simulink model "EPT"  (R2019b)
settings: Solver=FixedStepDiscrete  StartTime=0.0  StopTime=5  FixedStep=0.005  RelTol=1e-3  EnableMultiTasking=on
PreLoadFcn:
  | try, model_open; catch, disp('Error occurred while executing model pre-load callback: model_open.m'); disp('Please assure that the MATLAB working directory is set to the model directory before opening.'); end
InitFcn:
  | try, model_open; catch, end
undefined symbols (not defined in the file or in its folder): Bridge, GCM, H, ln, raptor_get_param_eval, raptor_get_safe_string, raptor_xcp_function
libraries: Raptor_lib x2810, simulink x374, hdlsllib x19
(part 30 of 45)

== system EPT/Foreground_TimeBase_5ms/CAN/CAN3_exec/HyPer9_MCU/TPDO2/Convert_Byte2Data3 ==
  LowByte : Inport
  HighByte : Inport  Port=2
  Offset : Inport  Port=3
  Factor : Inport  Port=4
  Add2 : Sum
  Add5 : Sum
  Compare To Zero : simulink/Logic and Bit Operations/Compare To Zero  relop===  OutDataTypeStr=boolean
  Constant1 : Constant
  Constant10 : Constant  Value=256
  Data Type Conversion1 : DataTypeConversion  OutDataTypeStr=int16
  Data Type Conversion10 : DataTypeConversion  OutDataTypeStr=double
  Divide6 : Product  Inputs=**
  Divide9 : Product  Inputs=**
  Switch : Switch  Criteria=u2 > Threshold
  Data : Outport  VectorParamsAs1DForOutWhenUnconnected=off
  wires:
  Constant1/1 -> Switch/1
  Factor/1 -> Compare To Zero/1, Switch/3
  Compare To Zero/1 -> Switch/2
  Switch/1 -> Divide9/2
  Divide6/1 -> Add2/2
  Add5/1 -> Data Type Conversion10/1
  Constant10/1 -> Divide6/2
  Divide9/1 -> Add5/1
  Add2/1 -> Data Type Conversion1/1
  Data Type Conversion10/1 -> Data/1
  Offset/1 -> Add5/2
  HighByte/1 -> Divide6/1
  LowByte/1 -> Add2/1
  Data Type Conversion1/1 -> Divide9/1

== system EPT/Foreground_TimeBase_5ms/CAN/CAN3_exec/HyPer9_MCU/TPDO3/Byte6 ==
  Byte : Inport
  Bitwise AND : simulink/Logic and Bit Operations/Bitwise Operator  logicop=AND  UseBitMask=on  BitMask=bin2dec('10')  BitMaskRealWorld=Stored Integer
  Bitwise AND1 : simulink/Logic and Bit Operations/Bitwise Operator  logicop=AND  UseBitMask=on  BitMask=bin2dec('100')  BitMaskRealWorld=Stored Integer
  Bitwise AND2 : simulink/Logic and Bit Operations/Bitwise Operator  logicop=AND  UseBitMask=on  BitMask=bin2dec('1000')  BitMaskRealWorld=Stored Integer
  Bitwise AND3 : simulink/Logic and Bit Operations/Bitwise Operator  logicop=AND  UseBitMask=on  BitMask=bin2dec('10000000')  BitMaskRealWorld=Stored Integer
  Bitwise AND7 : simulink/Logic and Bit Operations/Bitwise Operator  logicop=AND  UseBitMask=on  BitMask=bin2dec('1')  BitMaskRealWorld=Stored Integer
  IsPositive{,1..4} (5 alike) : simulink/Logic and Bit Operations/Compare To Zero  relop=>  OutDataTypeStr=boolean
  Digital Input 17 State : Outport
  Digital Input 18 State : Outport  Port=2
  Digital Input 19 State : Outport  Port=3
  "Toggle bit " : Outport  Port=4
  Driver Output 4 - State : Outport  Port=5
  wires:
  Bitwise AND7/1 -> IsPositive/1
  Bitwise AND3/1 -> IsPositive4/1
  Byte/1 -> Bitwise AND7/1, Bitwise AND1/1, Bitwise AND2/1, Bitwise AND3/1, Bitwise AND/1
  Bitwise AND/1 -> IsPositive1/1
  Bitwise AND2/1 -> IsPositive3/1
  Bitwise AND1/1 -> IsPositive2/1
  IsPositive/1 -> Digital Input 17 State/1
  IsPositive1/1 -> Digital Input 18 State/1
  IsPositive2/1 -> Digital Input 19 State/1
  IsPositive3/1 -> "Toggle bit "/1
  IsPositive4/1 -> Driver Output 4 - State/1

== system EPT/Foreground_TimeBase_5ms/CAN/CAN3_exec/HyPer9_MCU/TPDO3/Byte7 ==
  Byte : Inport
  Bit Shift : hdlsllib/Logic and Bit Operations/Bit Shift  mode=Shift Right Logical  N=5
  Bitwise AND : simulink/Logic and Bit Operations/Bitwise Operator  logicop=AND  UseBitMask=on  BitMask=bin2dec('10')  BitMaskRealWorld=Stored Integer
  Bitwise AND1 : simulink/Logic and Bit Operations/Bitwise Operator  logicop=AND  UseBitMask=on  BitMask=bin2dec('100')  BitMaskRealWorld=Stored Integer
  Bitwise AND2 : simulink/Logic and Bit Operations/Bitwise Operator  logicop=AND  UseBitMask=on  BitMask=bin2dec('1000')  BitMaskRealWorld=Stored Integer
  Bitwise AND3 : simulink/Logic and Bit Operations/Bitwise Operator  logicop=AND  UseBitMask=on  BitMask=bin2dec('10000')  BitMaskRealWorld=Stored Integer
  Bitwise AND4 : simulink/Logic and Bit Operations/Bitwise Operator  logicop=AND  UseBitMask=on  BitMask=bin2dec('11100000')  BitMaskRealWorld=Stored Integer
  Bitwise AND7 : simulink/Logic and Bit Operations/Bitwise Operator  logicop=AND  UseBitMask=on  BitMask=bin2dec('1')  BitMaskRealWorld=Stored Integer
  IsPositive{,1..4} (5 alike) : simulink/Logic and Bit Operations/Compare To Zero  relop=>  OutDataTypeStr=boolean
  Driver Output 1 - State : Outport
  Driver Output 2 - State : Outport  Port=2
  Driver Output 3 - State : Outport  Port=3
  Digital Output 1 - State : Outport  Port=4
  Digital Output 2 - State : Outport  Port=5
  "Fault Level " : Outport  Port=6
  wires:
  Bitwise AND1/1 -> IsPositive2/1
  Bitwise AND2/1 -> IsPositive3/1
  Bitwise AND/1 -> IsPositive1/1
  Bitwise AND4/1 -> Bit Shift/1
  Byte/1 -> Bitwise AND/1, Bitwise AND4/1, Bitwise AND3/1, Bitwise AND2/1, Bitwise AND1/1, Bitwise AND7/1
  Bitwise AND3/1 -> IsPositive4/1
  Bitwise AND7/1 -> IsPositive/1
  Bit Shift/1 -> "Fault Level "/1
  IsPositive/1 -> Driver Output 1 - State/1
  IsPositive1/1 -> Driver Output 2 - State/1
  IsPositive2/1 -> Driver Output 3 - State/1
  IsPositive3/1 -> Digital Output 1 - State/1
  IsPositive4/1 -> Digital Output 2 - State/1

== system EPT/Foreground_TimeBase_5ms/CAN/CAN3_exec/HyPer9_MCU/TPDO3/Convert_Byte2Data ==
  LowByte : Inport
  HighByte : Inport  Port=2
  Offset : Inport  Port=3
  Factor : Inport  Port=4
  Add2 : Sum
  Add5 : Sum
  Compare To Zero : simulink/Logic and Bit Operations/Compare To Zero  relop===  OutDataTypeStr=boolean
  Constant1 : Constant
  Constant10 : Constant  Value=256
  Data Type Conversion1 : DataTypeConversion  OutDataTypeStr=int16
  Data Type Conversion10 : DataTypeConversion  OutDataTypeStr=double
  Divide6 : Product  Inputs=**
  Divide9 : Product  Inputs=**
  Switch : Switch  Criteria=u2 > Threshold
  Data : Outport  VectorParamsAs1DForOutWhenUnconnected=off
  wires:
  Constant1/1 -> Switch/1
  Factor/1 -> Compare To Zero/1, Switch/3
  Compare To Zero/1 -> Switch/2
  Switch/1 -> Divide9/2
  Divide6/1 -> Add2/2
  Add5/1 -> Data Type Conversion10/1
  Constant10/1 -> Divide6/2
  Divide9/1 -> Add5/1
  Add2/1 -> Data Type Conversion1/1
  Data Type Conversion10/1 -> Data/1
  Offset/1 -> Add5/2
  HighByte/1 -> Divide6/1
  LowByte/1 -> Add2/1
  Data Type Conversion1/1 -> Divide9/1

== system EPT/Foreground_TimeBase_5ms/CAN/CAN3_exec/HyPer9_MCU/TPDO3/Convert_Byte2Data1 ==
  LowByte : Inport
  HighByte : Inport  Port=2
  Offset : Inport  Port=3
  Factor : Inport  Port=4
  Add2 : Sum
  Add5 : Sum
  Compare To Zero : simulink/Logic and Bit Operations/Compare To Zero  relop===  OutDataTypeStr=boolean
  Constant1 : Constant
  Constant10 : Constant  Value=256
  Data Type Conversion1 : DataTypeConversion  OutDataTypeStr=int16
  Data Type Conversion10 : DataTypeConversion  OutDataTypeStr=double
  Divide6 : Product  Inputs=**
  Divide9 : Product  Inputs=**
  Switch : Switch  Criteria=u2 > Threshold
  Data : Outport  VectorParamsAs1DForOutWhenUnconnected=off
  wires:
  Data Type Conversion1/1 -> Divide9/1
  LowByte/1 -> Add2/1
  HighByte/1 -> Divide6/1
  Offset/1 -> Add5/2
  Data Type Conversion10/1 -> Data/1
  Add2/1 -> Data Type Conversion1/1
  Divide9/1 -> Add5/1
  Constant10/1 -> Divide6/2
  Add5/1 -> Data Type Conversion10/1
  Divide6/1 -> Add2/2
  Switch/1 -> Divide9/2
  Compare To Zero/1 -> Switch/2
  Factor/1 -> Switch/3, Compare To Zero/1
  Constant1/1 -> Switch/1

== system EPT/Foreground_TimeBase_5ms/CAN/CAN3_exec/HyPer9_MCU/TPDO3/Digital Input 1 to 8 - State ==
  Byte : Inport
  Bitwise AND : simulink/Logic and Bit Operations/Bitwise Operator  logicop=AND  UseBitMask=on  BitMask=bin2dec('10')  BitMaskRealWorld=Stored Integer
  Bitwise AND1 : simulink/Logic and Bit Operations/Bitwise Operator  logicop=AND  UseBitMask=on  BitMask=bin2dec('100')  BitMaskRealWorld=Stored Integer
  Bitwise AND2 : simulink/Logic and Bit Operations/Bitwise Operator  logicop=AND  UseBitMask=on  BitMask=bin2dec('1000')  BitMaskRealWorld=Stored Integer
  Bitwise AND3 : simulink/Logic and Bit Operations/Bitwise Operator  logicop=AND  UseBitMask=on  BitMask=bin2dec('10000')  BitMaskRealWorld=Stored Integer
  Bitwise AND4 : simulink/Logic and Bit Operations/Bitwise Operator  logicop=AND  UseBitMask=on  BitMask=bin2dec('100000')  BitMaskRealWorld=Stored Integer
  Bitwise AND5 : simulink/Logic and Bit Operations/Bitwise Operator  logicop=AND  UseBitMask=on  BitMask=bin2dec('1000000')  BitMaskRealWorld=Stored Integer
  Bitwise AND6 : simulink/Logic and Bit Operations/Bitwise Operator  logicop=AND  UseBitMask=on  BitMask=bin2dec('10000000')  BitMaskRealWorld=Stored Integer
  Bitwise AND7 : simulink/Logic and Bit Operations/Bitwise Operator  logicop=AND  UseBitMask=on  BitMask=bin2dec('1')  BitMaskRealWorld=Stored Integer
  IsPositive{,1..7} (8 alike) : simulink/Logic and Bit Operations/Compare To Zero  relop=>  OutDataTypeStr=boolean
  Digital Input 1 State : Outport
  Digital Input 2 State : Outport  Port=2
  Digital Input 3 State : Outport  Port=3
  Digital Input 4 State : Outport  Port=4
  Digital Input 5 State : Outport  Port=5
  Digital Input 6 State : Outport  Port=6
  Digital Input 7 State : Outport  Port=7
  Digital Input 8 State : Outport  Port=8
  wires:
  Bitwise AND1/1 -> IsPositive2/1
  Bitwise AND2/1 -> IsPositive3/1
  Bitwise AND/1 -> IsPositive1/1
  Bitwise AND4/1 -> IsPositive5/1
  Byte/1 -> Bitwise AND/1, Bitwise AND6/1, Bitwise AND5/1, Bitwise AND4/1, Bitwise AND3/1, Bitwise AND2/1, Bitwise AND1/1, Bitwise AND7/1
  Bitwise AND3/1 -> IsPositive4/1
  Bitwise AND6/1 -> IsPositive7/1
  Bitwise AND5/1 -> IsPositive6/1
  Bitwise AND7/1 -> IsPositive/1
  IsPositive/1 -> Digital Input 1 State/1
  IsPositive1/1 -> Digital Input 2 State/1
  IsPositive2/1 -> Digital Input 3 State/1
  IsPositive3/1 -> Digital Input 4 State/1
  IsPositive4/1 -> Digital Input 5 State/1
  IsPositive5/1 -> Digital Input 6 State/1
  IsPositive6/1 -> Digital Input 7 State/1
  IsPositive7/1 -> Digital Input 8 State/1

== system EPT/Foreground_TimeBase_5ms/CAN/CAN3_exec/HyPer9_MCU/TPDO3/Digital Input 9 to 16 - State ==
  Byte : Inport
  Bitwise AND : simulink/Logic and Bit Operations/Bitwise Operator  logicop=AND  UseBitMask=on  BitMask=bin2dec('10')  BitMaskRealWorld=Stored Integer
  Bitwise AND1 : simulink/Logic and Bit Operations/Bitwise Operator  logicop=AND  UseBitMask=on  BitMask=bin2dec('100')  BitMaskRealWorld=Stored Integer
  Bitwise AND2 : simulink/Logic and Bit Operations/Bitwise Operator  logicop=AND  UseBitMask=on  BitMask=bin2dec('1000')  BitMaskRealWorld=Stored Integer
  Bitwise AND3 : simulink/Logic and Bit Operations/Bitwise Operator  logicop=AND  UseBitMask=on  BitMask=bin2dec('10000')  BitMaskRealWorld=Stored Integer
  Bitwise AND4 : simulink/Logic and Bit Operations/Bitwise Operator  logicop=AND  UseBitMask=on  BitMask=bin2dec('100000')  BitMaskRealWorld=Stored Integer
  Bitwise AND5 : simulink/Logic and Bit Operations/Bitwise Operator  logicop=AND  UseBitMask=on  BitMask=bin2dec('1000000')  BitMaskRealWorld=Stored Integer
  Bitwise AND6 : simulink/Logic and Bit Operations/Bitwise Operator  logicop=AND  UseBitMask=on  BitMask=bin2dec('10000000')  BitMaskRealWorld=Stored Integer
  Bitwise AND7 : simulink/Logic and Bit Operations/Bitwise Operator  logicop=AND  UseBitMask=on  BitMask=bin2dec('1')  BitMaskRealWorld=Stored Integer
  IsPositive{,1..7} (8 alike) : simulink/Logic and Bit Operations/Compare To Zero  relop=>  OutDataTypeStr=boolean
  Digital Input 9 State : Outport
  Digital Input 10 State : Outport  Port=2
  Digital Input 11 State : Outport  Port=3
  Digital Input 12 State : Outport  Port=4
  Digital Input 13 State : Outport  Port=5
  Digital Input 14 State : Outport  Port=6
  Digital Input 15 State : Outport  Port=7
  Digital Input 16 State : Outport  Port=8
  wires:
  Bitwise AND7/1 -> IsPositive/1
  Bitwise AND5/1 -> IsPositive6/1
  Bitwise AND6/1 -> IsPositive7/1
  Bitwise AND3/1 -> IsPositive4/1
  Byte/1 -> Bitwise AND7/1, Bitwise AND1/1, Bitwise AND2/1, Bitwise AND3/1, Bitwise AND4/1, Bitwise AND5/1, Bitwise AND6/1, Bitwise AND/1
  Bitwise AND4/1 -> IsPositive5/1
  Bitwise AND/1 -> IsPositive1/1
  Bitwise AND2/1 -> IsPositive3/1
  Bitwise AND1/1 -> IsPositive2/1
  IsPositive/1 -> Digital Input 9 State/1
  IsPositive1/1 -> Digital Input 10 State/1
  IsPositive2/1 -> Digital Input 11 State/1
  IsPositive3/1 -> Digital Input 12 State/1
  IsPositive4/1 -> Digital Input 13 State/1
  IsPositive5/1 -> Digital Input 14 State/1
  IsPositive6/1 -> Digital Input 15 State/1
  IsPositive7/1 -> Digital Input 16 State/1

== system EPT/Foreground_TimeBase_5ms/CAN/CAN3_exec/HyPer9_MCU/TPDO4/Byte6 ==
  Byte : Inport
  Bitwise AND : simulink/Logic and Bit Operations/Bitwise Operator  logicop=AND  UseBitMask=on  BitMask=bin2dec('100')  BitMaskRealWorld=Stored Integer
  Bitwise AND1 : simulink/Logic and Bit Operations/Bitwise Operator  logicop=AND  UseBitMask=on  BitMask=bin2dec('1000')  BitMaskRealWorld=Stored Integer
  Bitwise AND2 : simulink/Logic and Bit Operations/Bitwise Operator  logicop=AND  UseBitMask=on  BitMask=bin2dec('10000')  BitMaskRealWorld=Stored Integer
  Bitwise AND3 : simulink/Logic and Bit Operations/Bitwise Operator  logicop=AND  UseBitMask=on  BitMask=bin2dec('100000')  BitMaskRealWorld=Stored Integer
  Bitwise AND4 : simulink/Logic and Bit Operations/Bitwise Operator  logicop=AND  UseBitMask=on  BitMask=bin2dec('1000000')  BitMaskRealWorld=Stored Integer
  Bitwise AND7 : simulink/Logic and Bit Operations/Bitwise Operator  logicop=AND  UseBitMask=on  BitMask=bin2dec('11')  BitMaskRealWorld=Stored Integer
  IsPositive{1..5} (5 alike) : simulink/Logic and Bit Operations/Compare To Zero  relop=>  OutDataTypeStr=boolean
  Motor 1 - Control Mode : Outport
  Motor 1 - PWM Output : Outport  Port=2
  Motor 1 - Reference Speed/Torque : Outport  Port=3
  Motor 1 - Emergency Stop : Outport  Port=4
  Motor 1 - Safe Stop : Outport  Port=5
  Motor 1 - Speed Limit : Outport  Port=6
  wires:
  IsPositive4/1 -> Motor 1 - Safe Stop/1
  IsPositive3/1 -> Motor 1 - Emergency Stop/1
  IsPositive2/1 -> Motor 1 - Reference Speed/Torque/1
  IsPositive1/1 -> Motor 1 - PWM Output/1
  Bitwise AND7/1 -> Motor 1 - Control Mode/1
  Bitwise AND1/1 -> IsPositive2/1
  Bitwise AND2/1 -> IsPositive3/1
  Bitwise AND/1 -> IsPositive1/1
  Byte/1 -> Bitwise AND/1, Bitwise AND4/1, Bitwise AND3/1, Bitwise AND2/1, Bitwise AND1/1, Bitwise AND7/1
  Bitwise AND3/1 -> IsPositive4/1
  Bitwise AND4/1 -> IsPositive5/1
  IsPositive5/1 -> Motor 1 - Speed Limit/1

== system EPT/Foreground_TimeBase_5ms/CAN/CAN3_exec/HyPer9_MCU/TPDO4/Convert_Byte2Data ==
  LowByte : Inport
  HighByte : Inport  Port=2
  Offset : Inport  Port=3
  Factor : Inport  Port=4
  Add2 : Sum
  Add5 : Sum
  Compare To Zero : simulink/Logic and Bit Operations/Compare To Zero  relop===  OutDataTypeStr=boolean
  Constant1 : Constant
  Constant10 : Constant  Value=256
  Data Type Conversion1 : DataTypeConversion  OutDataTypeStr=int16
  Data Type Conversion10 : DataTypeConversion  OutDataTypeStr=double
  Divide6 : Product  Inputs=**
  Divide9 : Product  Inputs=**
  Switch : Switch  Criteria=u2 > Threshold
  Data : Outport  VectorParamsAs1DForOutWhenUnconnected=off
  wires:
  Data Type Conversion1/1 -> Divide9/1
  LowByte/1 -> Add2/1
  HighByte/1 -> Divide6/1
  Offset/1 -> Add5/2
  Data Type Conversion10/1 -> Data/1
  Add2/1 -> Data Type Conversion1/1
  Divide9/1 -> Add5/1
  Constant10/1 -> Divide6/2
  Add5/1 -> Data Type Conversion10/1
  Divide6/1 -> Add2/2
  Switch/1 -> Divide9/2
  Compare To Zero/1 -> Switch/2
  Factor/1 -> Switch/3, Compare To Zero/1
  Constant1/1 -> Switch/1

== system EPT/Foreground_TimeBase_5ms/CAN/CAN3_exec/HyPer9_MCU/TPDO4/Convert_Byte2Data1 ==
  LowByte : Inport
  HighByte : Inport  Port=2
  Offset : Inport  Port=3
  Factor : Inport  Port=4
  Add2 : Sum
  Add5 : Sum
  Compare To Zero : simulink/Logic and Bit Operations/Compare To Zero  relop===  OutDataTypeStr=boolean
  Constant1 : Constant
  Constant10 : Constant  Value=256
  Data Type Conversion1 : DataTypeConversion  OutDataTypeStr=int16
  Data Type Conversion10 : DataTypeConversion  OutDataTypeStr=double
  Divide6 : Product  Inputs=**
  Divide9 : Product  Inputs=**
  Switch : Switch  Criteria=u2 > Threshold
  Data : Outport  VectorParamsAs1DForOutWhenUnconnected=off
  wires:
  Constant1/1 -> Switch/1
  Factor/1 -> Compare To Zero/1, Switch/3
  Compare To Zero/1 -> Switch/2
  Switch/1 -> Divide9/2
  Divide6/1 -> Add2/2
  Add5/1 -> Data Type Conversion10/1
  Constant10/1 -> Divide6/2
  Divide9/1 -> Add5/1
  Add2/1 -> Data Type Conversion1/1
  Data Type Conversion10/1 -> Data/1
  Offset/1 -> Add5/2
  HighByte/1 -> Divide6/1
  LowByte/1 -> Add2/1
  Data Type Conversion1/1 -> Divide9/1

== system EPT/Foreground_TimeBase_5ms/CAN/CAN3_exec/HyPer9_MCU/TPDO4/Convert_Byte2Data2 ==
  Offset : Inport
  LowByte : Inport  Port=2
  Factor : Inport  Port=3
  Add5 : Sum
  Compare To Zero : simulink/Logic and Bit Operations/Compare To Zero  relop===  OutDataTypeStr=boolean
  Constant1 : Constant
  Data Type Conversion1 : DataTypeConversion  OutDataTypeStr=uint8
  Data Type Conversion10 : DataTypeConversion  OutDataTypeStr=double
  Divide9 : Product  Inputs=**
  Switch : Switch  Criteria=u2 > Threshold
  Data : Outport  VectorParamsAs1DForOutWhenUnconnected=off
  wires:
  Data Type Conversion10/1 -> Data/1
  Offset/1 -> Add5/2
  Compare To Zero/1 -> Switch/2
  Data Type Conversion1/1 -> Divide9/1
  Add5/1 -> Data Type Conversion10/1
  Divide9/1 -> Add5/1
  Switch/1 -> Divide9/2
  Constant1/1 -> Switch/1
  Factor/1 -> Compare To Zero/1, Switch/3
  LowByte/1 -> Data Type Conversion1/1

== system EPT/Foreground_TimeBase_5ms/CAN/CAN3_exec/HyPer9_MCU/TPDO4/Convert_Byte2Data3 ==
  Offset : Inport
  LowByte : Inport  Port=2
  Factor : Inport  Port=3
  Add5 : Sum
  Compare To Zero : simulink/Logic and Bit Operations/Compare To Zero  relop===  OutDataTypeStr=boolean
  Constant1 : Constant
  Data Type Conversion1 : DataTypeConversion  OutDataTypeStr=uint8
  Data Type Conversion10 : DataTypeConversion  OutDataTypeStr=double
  Divide9 : Product  Inputs=**
  Switch : Switch  Criteria=u2 > Threshold
  Data : Outport  VectorParamsAs1DForOutWhenUnconnected=off
  wires:
  LowByte/1 -> Data Type Conversion1/1
  Factor/1 -> Switch/3, Compare To Zero/1
  Constant1/1 -> Switch/1
  Switch/1 -> Divide9/2
  Divide9/1 -> Add5/1
  Add5/1 -> Data Type Conversion10/1
  Data Type Conversion1/1 -> Divide9/1
  Compare To Zero/1 -> Switch/2
  Offset/1 -> Add5/2
  Data Type Conversion10/1 -> Data/1

== system EPT/Foreground_TimeBase_5ms/CAN/CAN3_exec/HyPer9_MCU/TPDO4/Motor 1 - State ==
  Byte : Inport
  Bitwise AND7 : simulink/Logic and Bit Operations/Bitwise Operator  logicop=AND  UseBitMask=on  BitMask=bin2dec('1111')  BitMaskRealWorld=Stored Integer
  Motor 1 - State : Outport
  wires:
  Bitwise AND7/1 -> Motor 1 - State/1
  Byte/1 -> Bitwise AND7/1

== system EPT/Foreground_TimeBase_5ms/CAN/CAN3_exec/HyPer9_MCU/TPDO5/Byte6 ==
  Byte : Inport
  Bitwise AND : simulink/Logic and Bit Operations/Bitwise Operator  logicop=AND  UseBitMask=on  BitMask=bin2dec('100')  BitMaskRealWorld=Stored Integer
  Bitwise AND1 : simulink/Logic and Bit Operations/Bitwise Operator  logicop=AND  UseBitMask=on  BitMask=bin2dec('1000')  BitMaskRealWorld=Stored Integer
  Bitwise AND2 : simulink/Logic and Bit Operations/Bitwise Operator  logicop=AND  UseBitMask=on  BitMask=bin2dec('10000')  BitMaskRealWorld=Stored Integer
  Bitwise AND3 : simulink/Logic and Bit Operations/Bitwise Operator  logicop=AND  UseBitMask=on  BitMask=bin2dec('100000')  BitMaskRealWorld=Stored Integer
  Bitwise AND4 : simulink/Logic and Bit Operations/Bitwise Operator  logicop=AND  UseBitMask=on  BitMask=bin2dec('1000000')  BitMaskRealWorld=Stored Integer
  Bitwise AND7 : simulink/Logic and Bit Operations/Bitwise Operator  logicop=AND  UseBitMask=on  BitMask=bin2dec('11')  BitMaskRealWorld=Stored Integer
  IsPositive{1..5} (5 alike) : simulink/Logic and Bit Operations/Compare To Zero  relop=>  OutDataTypeStr=boolean
  Motor 2 - Control Mode : Outport
  Motor 2 - PWM Output : Outport  Port=2
  Motor 2 - Reference Speed/Torque : Outport  Port=3
  Motor 2 - Emergency Stop : Outport  Port=4
  Motor 2 - Safe Stop : Outport  Port=5
  Motor 2 - Speed Limit : Outport  Port=6
  wires:
  IsPositive5/1 -> Motor 2 - Speed Limit/1
  Bitwise AND4/1 -> IsPositive5/1
  Bitwise AND3/1 -> IsPositive4/1
  Byte/1 -> Bitwise AND7/1, Bitwise AND1/1, Bitwise AND2/1, Bitwise AND3/1, Bitwise AND4/1, Bitwise AND/1
  Bitwise AND/1 -> IsPositive1/1
  Bitwise AND2/1 -> IsPositive3/1
  Bitwise AND1/1 -> IsPositive2/1
  Bitwise AND7/1 -> Motor 2 - Control Mode/1
  IsPositive1/1 -> Motor 2 - PWM Output/1
  IsPositive2/1 -> Motor 2 - Reference Speed/Torque/1
  IsPositive3/1 -> Motor 2 - Emergency Stop/1
  IsPositive4/1 -> Motor 2 - Safe Stop/1

== system EPT/Foreground_TimeBase_5ms/CAN/CAN3_exec/HyPer9_MCU/TPDO5/Byte7 ==
  Byte : Inport
  Bitwise AND7 : simulink/Logic and Bit Operations/Bitwise Operator  logicop=AND  UseBitMask=on  BitMask=bin2dec('1111')  BitMaskRealWorld=Stored Integer
  Motor 2 - State : Outport
  wires:
  Byte/1 -> Bitwise AND7/1
  Bitwise AND7/1 -> Motor 2 - State/1

== system EPT/Foreground_TimeBase_5ms/CAN/CAN3_exec/HyPer9_MCU/TPDO5/Convert_Byte2Data ==
  LowByte : Inport
  HighByte : Inport  Port=2
  Offset : Inport  Port=3
  Factor : Inport  Port=4
  Add2 : Sum
  Add5 : Sum
  Compare To Zero : simulink/Logic and Bit Operations/Compare To Zero  relop===  OutDataTypeStr=boolean
  Constant1 : Constant
  Constant10 : Constant  Value=256
  Data Type Conversion1 : DataTypeConversion  OutDataTypeStr=int16
  Data Type Conversion10 : DataTypeConversion  OutDataTypeStr=double
  Divide6 : Product  Inputs=**
  Divide9 : Product  Inputs=**
  Switch : Switch  Criteria=u2 > Threshold
  Data : Outport  VectorParamsAs1DForOutWhenUnconnected=off
  wires:
  Constant1/1 -> Switch/1
  Factor/1 -> Compare To Zero/1, Switch/3
  Compare To Zero/1 -> Switch/2
  Switch/1 -> Divide9/2
  Divide6/1 -> Add2/2
  Add5/1 -> Data Type Conversion10/1
  Constant10/1 -> Divide6/2
  Divide9/1 -> Add5/1
  Add2/1 -> Data Type Conversion1/1
  Data Type Conversion10/1 -> Data/1
  Offset/1 -> Add5/2
  HighByte/1 -> Divide6/1
  LowByte/1 -> Add2/1
  Data Type Conversion1/1 -> Divide9/1

== system EPT/Foreground_TimeBase_5ms/CAN/CAN3_exec/HyPer9_MCU/TPDO5/Convert_Byte2Data1 ==
  LowByte : Inport
  HighByte : Inport  Port=2
  Offset : Inport  Port=3
  Factor : Inport  Port=4
  Add2 : Sum
  Add5 : Sum
  Compare To Zero : simulink/Logic and Bit Operations/Compare To Zero  relop===  OutDataTypeStr=boolean
  Constant1 : Constant
  Constant10 : Constant  Value=256
  Data Type Conversion1 : DataTypeConversion  OutDataTypeStr=int16
  Data Type Conversion10 : DataTypeConversion  OutDataTypeStr=double
  Divide6 : Product  Inputs=**
  Divide9 : Product  Inputs=**
  Switch : Switch  Criteria=u2 > Threshold
  Data : Outport  VectorParamsAs1DForOutWhenUnconnected=off
  wires:
  Data Type Conversion1/1 -> Divide9/1
  LowByte/1 -> Add2/1
  HighByte/1 -> Divide6/1
  Offset/1 -> Add5/2
  Data Type Conversion10/1 -> Data/1
  Add2/1 -> Data Type Conversion1/1
  Divide9/1 -> Add5/1
  Constant10/1 -> Divide6/2
  Add5/1 -> Data Type Conversion10/1
  Divide6/1 -> Add2/2
  Switch/1 -> Divide9/2
  Compare To Zero/1 -> Switch/2
  Factor/1 -> Switch/3, Compare To Zero/1
  Constant1/1 -> Switch/1

== system EPT/Foreground_TimeBase_5ms/CAN/CAN3_exec/HyPer9_MCU/TPDO5/Convert_Byte2Data2 ==
  Offset : Inport
  LowByte : Inport  Port=2
  Factor : Inport  Port=3
  Add5 : Sum
  Compare To Zero : simulink/Logic and Bit Operations/Compare To Zero  relop===  OutDataTypeStr=boolean
  Constant1 : Constant
  Data Type Conversion1 : DataTypeConversion  OutDataTypeStr=uint8
  Data Type Conversion10 : DataTypeConversion  OutDataTypeStr=double
  Divide9 : Product  Inputs=**
  Switch : Switch  Criteria=u2 > Threshold
  Data : Outport  VectorParamsAs1DForOutWhenUnconnected=off
  wires:
  LowByte/1 -> Data Type Conversion1/1
  Factor/1 -> Switch/3, Compare To Zero/1
  Constant1/1 -> Switch/1
  Switch/1 -> Divide9/2
  Divide9/1 -> Add5/1
  Add5/1 -> Data Type Conversion10/1
  Data Type Conversion1/1 -> Divide9/1
  Compare To Zero/1 -> Switch/2
  Offset/1 -> Add5/2
  Data Type Conversion10/1 -> Data/1

== system EPT/Foreground_TimeBase_5ms/CAN/CAN3_exec/HyPer9_MCU/TPDO5/Convert_Byte2Data3 ==
  Offset : Inport
  LowByte : Inport  Port=2
  Factor : Inport  Port=3
  Add5 : Sum
  Compare To Zero : simulink/Logic and Bit Operations/Compare To Zero  relop===  OutDataTypeStr=boolean
  Constant1 : Constant
  Data Type Conversion1 : DataTypeConversion  OutDataTypeStr=uint8
  Data Type Conversion10 : DataTypeConversion  OutDataTypeStr=double
  Divide9 : Product  Inputs=**
  Switch : Switch  Criteria=u2 > Threshold
  Data : Outport  VectorParamsAs1DForOutWhenUnconnected=off
  wires:
  Data Type Conversion10/1 -> Data/1
  Offset/1 -> Add5/2
  Compare To Zero/1 -> Switch/2
  Data Type Conversion1/1 -> Divide9/1
  Add5/1 -> Data Type Conversion10/1
  Divide9/1 -> Add5/1
  Switch/1 -> Divide9/2
  Constant1/1 -> Switch/1
  Factor/1 -> Compare To Zero/1, Switch/3
  LowByte/1 -> Data Type Conversion1/1

== system EPT/Foreground_TimeBase_5ms/CAN/CAN3_exec/HyPer9_MCU/TPDO6/Convert_Byte2Data ==
  LowByte : Inport
  HighByte : Inport  Port=2
  Offset : Inport  Port=3
  Factor : Inport  Port=4
  Add2 : Sum
  Add5 : Sum
  Compare To Zero : simulink/Logic and Bit Operations/Compare To Zero  relop===  OutDataTypeStr=boolean
  Constant1 : Constant
  Constant10 : Constant  Value=256
  Data Type Conversion1 : DataTypeConversion  OutDataTypeStr=int16
  Data Type Conversion10 : DataTypeConversion  OutDataTypeStr=double
  Divide6 : Product  Inputs=**
  Divide9 : Product  Inputs=**
  Switch : Switch  Criteria=u2 > Threshold
  Data : Outport  VectorParamsAs1DForOutWhenUnconnected=off
  wires:
  Data Type Conversion1/1 -> Divide9/1
  LowByte/1 -> Add2/1
  HighByte/1 -> Divide6/1
  Offset/1 -> Add5/2
  Data Type Conversion10/1 -> Data/1
  Add2/1 -> Data Type Conversion1/1
  Divide9/1 -> Add5/1
  Constant10/1 -> Divide6/2
  Add5/1 -> Data Type Conversion10/1
  Divide6/1 -> Add2/2
  Switch/1 -> Divide9/2
  Compare To Zero/1 -> Switch/2
  Factor/1 -> Switch/3, Compare To Zero/1
  Constant1/1 -> Switch/1

== system EPT/Foreground_TimeBase_5ms/CAN/CAN3_exec/HyPer9_MCU/TPDO6/Convert_Byte2Data1 ==
  LowByte : Inport
  HighByte : Inport  Port=2
  Offset : Inport  Port=3
  Factor : Inport  Port=4
  Add2 : Sum
  Add5 : Sum
  Compare To Zero : simulink/Logic and Bit Operations/Compare To Zero  relop===  OutDataTypeStr=boolean
  Constant1 : Constant
  Constant10 : Constant  Value=256
  Data Type Conversion1 : DataTypeConversion  OutDataTypeStr=int16
  Data Type Conversion10 : DataTypeConversion  OutDataTypeStr=double
  Divide6 : Product  Inputs=**
  Divide9 : Product  Inputs=**
  Switch : Switch  Criteria=u2 > Threshold
  Data : Outport  VectorParamsAs1DForOutWhenUnconnected=off
  wires:
  Constant1/1 -> Switch/1
  Factor/1 -> Compare To Zero/1, Switch/3
  Compare To Zero/1 -> Switch/2
  Switch/1 -> Divide9/2
  Divide6/1 -> Add2/2
  Add5/1 -> Data Type Conversion10/1
  Constant10/1 -> Divide6/2
  Divide9/1 -> Add5/1
  Add2/1 -> Data Type Conversion1/1
  Data Type Conversion10/1 -> Data/1
  Offset/1 -> Add5/2
  HighByte/1 -> Divide6/1
  LowByte/1 -> Add2/1
  Data Type Conversion1/1 -> Divide9/1

== system EPT/Foreground_TimeBase_5ms/CAN/CAN3_exec/HyPer9_MCU/TPDO6/Convert_Byte2Data2 ==
  LowByte : Inport
  HighByte : Inport  Port=2
  Offset : Inport  Port=3
  Factor : Inport  Port=4
  Add2 : Sum
  Add5 : Sum
  Compare To Zero : simulink/Logic and Bit Operations/Compare To Zero  relop===  OutDataTypeStr=boolean
  Constant1 : Constant
  Constant10 : Constant  Value=256
  Data Type Conversion1 : DataTypeConversion  OutDataTypeStr=int16
  Data Type Conversion10 : DataTypeConversion  OutDataTypeStr=double
  Divide6 : Product  Inputs=**
  Divide9 : Product  Inputs=**
  Switch : Switch  Criteria=u2 > Threshold
  Data : Outport  VectorParamsAs1DForOutWhenUnconnected=off
  wires:
  Data Type Conversion1/1 -> Divide9/1
  LowByte/1 -> Add2/1
  HighByte/1 -> Divide6/1
  Offset/1 -> Add5/2
  Data Type Conversion10/1 -> Data/1
  Add2/1 -> Data Type Conversion1/1
  Divide9/1 -> Add5/1
  Constant10/1 -> Divide6/2
  Add5/1 -> Data Type Conversion10/1
  Divide6/1 -> Add2/2
  Switch/1 -> Divide9/2
  Compare To Zero/1 -> Switch/2
  Factor/1 -> Switch/3, Compare To Zero/1
  Constant1/1 -> Switch/1

== system EPT/Foreground_TimeBase_5ms/CAN/CAN3_exec/HyPer9_MCU/TPDO6/Convert_Byte2Data3 ==
  Offset : Inport
  LowByte : Inport  Port=2
  Factor : Inport  Port=3
  Add5 : Sum
  Compare To Zero : simulink/Logic and Bit Operations/Compare To Zero  relop===  OutDataTypeStr=boolean
  Constant1 : Constant
  Data Type Conversion1 : DataTypeConversion  OutDataTypeStr=uint8
  Data Type Conversion10 : DataTypeConversion  OutDataTypeStr=double
  Divide9 : Product  Inputs=**
  Switch : Switch  Criteria=u2 > Threshold
  Data : Outport  VectorParamsAs1DForOutWhenUnconnected=off
  wires:
  Data Type Conversion10/1 -> Data/1
  Offset/1 -> Add5/2
  Compare To Zero/1 -> Switch/2
  Data Type Conversion1/1 -> Divide9/1
  Add5/1 -> Data Type Conversion10/1
  Divide9/1 -> Add5/1
  Switch/1 -> Divide9/2
  Constant1/1 -> Switch/1
  Factor/1 -> Compare To Zero/1, Switch/3
  LowByte/1 -> Data Type Conversion1/1

== system EPT/Foreground_TimeBase_5ms/CAN/CAN3_exec/HyPer9_MCU/TPDO6/Convert_Byte2Data4 ==
  Offset : Inport
  LowByte : Inport  Port=2
  Factor : Inport  Port=3
  Add5 : Sum
  Compare To Zero : simulink/Logic and Bit Operations/Compare To Zero  relop===  OutDataTypeStr=boolean
  Constant1 : Constant
  Data Type Conversion1 : DataTypeConversion  OutDataTypeStr=uint8
  Data Type Conversion10 : DataTypeConversion  OutDataTypeStr=double
  Divide9 : Product  Inputs=**
  Switch : Switch  Criteria=u2 > Threshold
  Data : Outport  VectorParamsAs1DForOutWhenUnconnected=off
  wires:
  LowByte/1 -> Data Type Conversion1/1
  Factor/1 -> Switch/3, Compare To Zero/1
  Constant1/1 -> Switch/1
  Switch/1 -> Divide9/2
  Divide9/1 -> Add5/1
  Add5/1 -> Data Type Conversion10/1
  Data Type Conversion1/1 -> Divide9/1
  Compare To Zero/1 -> Switch/2
  Offset/1 -> Add5/2
  Data Type Conversion10/1 -> Data/1

== system EPT/Foreground_TimeBase_5ms/CAN/CAN3_exec/OBC/CountTrigger/CycleTrigger ==
  In1 : Inport
  In2 : Inport  Port=2
  Add : Sum
  Add1 : Sum
  Add2 : Sum  Inputs=+-
  Constant1 : Constant
  Constant2 : Constant  Value=0
  Constant3 : Constant
  Data Type Conversion1 : DataTypeConversion
  Data Type Conversion2 : DataTypeConversion
  Display : Display
  Relational Operator1 : RelationalOperator  OutDataTypeStr=boolean  RndMeth=Simplest
  Scope : Scope
  Scope1 : Scope
  Scope2 : Scope
  Switch : Switch  Threshold=1
  Unit Delay : UnitDelay  SampleTime=-1  HasFrameUpgradeWarning=on
  Unit Delay1 : UnitDelay  SampleTime=-1  HasFrameUpgradeWarning=on
  Trigger : Outport  VectorParamsAs1DForOutWhenUnconnected=off
  wires:
  Add/1 -> Switch/1
  In1/1 -> Data Type Conversion2/1
  Unit Delay/1 -> Add/1
  Switch/1 -> Relational Operator1/1, Scope1/1, Unit Delay/1
  Add1/1 -> Scope/1, Unit Delay1/1, Display/1
  Unit Delay1/1 -> Add1/1
  Constant1/1 -> Add1/2
  Relational Operator1/1 -> Scope2/1, Trigger/1
  Data Type Conversion1/1 -> Relational Operator1/2
  Constant2/1 -> Switch/3
  Data Type Conversion2/1 -> Add/2, Switch/2
  Add2/1 -> Data Type Conversion1/1
  In2/1 -> Add2/1
  Constant3/1 -> Add2/2

== system EPT/Foreground_TimeBase_5ms/CAN/CAN3_exec/OBC/CountTrigger1/CycleTrigger ==
  In1 : Inport
  In2 : Inport  Port=2
  Add : Sum
  Add1 : Sum
  Add2 : Sum  Inputs=+-
  Constant1 : Constant
  Constant2 : Constant  Value=0
  Constant3 : Constant
  Data Type Conversion1 : DataTypeConversion
  Data Type Conversion2 : DataTypeConversion
  Display : Display
  Relational Operator1 : RelationalOperator  OutDataTypeStr=boolean  RndMeth=Simplest
  Scope : Scope
  Scope1 : Scope
  Scope2 : Scope
  Switch : Switch  Threshold=1
  Unit Delay : UnitDelay  SampleTime=-1  HasFrameUpgradeWarning=on
  Unit Delay1 : UnitDelay  SampleTime=-1  HasFrameUpgradeWarning=on
  Trigger : Outport  VectorParamsAs1DForOutWhenUnconnected=off
  wires:
  Add/1 -> Switch/1
  In1/1 -> Data Type Conversion2/1
  Unit Delay/1 -> Add/1
  Switch/1 -> Relational Operator1/1, Scope1/1, Unit Delay/1
  Add1/1 -> Scope/1, Unit Delay1/1, Display/1
  Unit Delay1/1 -> Add1/1
  Constant1/1 -> Add1/2
  Relational Operator1/1 -> Scope2/1, Trigger/1
  Data Type Conversion1/1 -> Relational Operator1/2
  Constant2/1 -> Switch/3
  Data Type Conversion2/1 -> Add/2, Switch/2
  Add2/1 -> Data Type Conversion1/1
  In2/1 -> Add2/1
  Constant3/1 -> Add2/2

== system EPT/Foreground_TimeBase_5ms/CAN/CAN3_exec/OBC/OBC/OBC_Rx ==
  note: PA2-1 0x180150E5
      | PA2-2 0x18FF50E5
      | PA2-3 0x18FF50E5
  Trigger : TriggerPort  VariantControl=Variant  PortDimensions=1
  Constant : Constant  Value=0.1
  Constant1 : Constant  Value=-40
  Constant2 : Constant
  Convert_Byte2Data1 : Subsystem
  Convert_Byte2Data2 : Subsystem
  Convert_Byte2Data3 : Subsystem
  Data Type Conversion : DataTypeConversion
  Data Type Conversion1 : DataTypeConversion  OutDataTypeStr=double
  Demux : Demux  Outputs=8
  Demux1 : Demux
  Mux : Mux
  raptor_can_rxraw : Raptor_lib/CAN/raptor_can_rxraw  canBus='CAN3'  extendedId=1  showAge=1  id=hex2dec('18FF50E5')  idMask=hex2dec('1F00FFFF')  mailbox=''  queueSize=15
      settings: SourceProductName=Raptor
  raptor_data_def : Raptor_lib/Data Storage/raptor_data_def  dataName='OBC_Age'  initValue=0  dataType=uint16  storage=Volatile (RAM)  calVisible=on  calType=Measurement  calDispType=Number  calEnum={'False', 'True'}  calGain=1.0  calOffset=0  calMin=-inf  calMax=inf  calFormat='-1'  calUnit=''  calHelp=''  calAccess=1  calFunction=raptor_xcp_function(gcb)  calDispHeaders=off  calColHeaders={'Col1' 'Col2' 'Col3'}  calRowHeaders={'Row1' 'Row2' 'Row3'}
      settings: SourceProductName=Raptor
  raptor_data_def1 : Raptor_lib/Data Storage/raptor_data_def  dataName='Read_OBC_Status'  initValue=0  dataType=uint8  storage=Volatile (RAM)  calVisible=on  calType=Measurement  calDispType=Number  calEnum={'False', 'True'}  calGain=1.0  calOffset=0  calMin=-inf  calMax=inf  calFormat='-1'  calUnit=''  calHelp=''  calAccess=1  calFunction=raptor_xcp_function(gcb)  calDispHeaders=off  calColHeaders={'Col1' 'Col2' 'Col3'}  calRowHeaders={'Row1' 'Row2' 'Row3'}
      settings: SourceProductName=Raptor
  raptor_data_def2 : Raptor_lib/Data Storage/raptor_data_def  dataName='Read_OBC_Cout'  initValue=0  dataType=double  storage=Volatile (RAM)  calVisible=on  calType=Measurement  calDispType=Number  calEnum={'False', 'True'}  calGain=1.0  calOffset=0  calMin=-inf  calMax=inf  calFormat='-1'  calUnit=''  calHelp=''  calAccess=1  calFunction=raptor_xcp_function(gcb)  calDispHeaders=off  calColHeaders={'Col1' 'Col2' 'Col3'}  calRowHeaders={'Row1' 'Row2' 'Row3'}
      settings: SourceProductName=Raptor
  raptor_data_def3 : Raptor_lib/Data Storage/raptor_data_def  dataName='Read_OBC_Vout'  initValue=0  dataType=double  storage=Volatile (RAM)  calVisible=on  calType=Measurement  calDispType=Number  calEnum={'False', 'True'}  calGain=1.0  calOffset=0  calMin=-inf  calMax=inf  calFormat='-1'  calUnit=''  calHelp=''  calAccess=1  calFunction=raptor_xcp_function(gcb)  calDispHeaders=off  calColHeaders={'Col1' 'Col2' 'Col3'}  calRowHeaders={'Row1' 'Row2' 'Row3'}
      settings: SourceProductName=Raptor
  raptor_data_def4 : Raptor_lib/Data Storage/raptor_data_def  dataName='Read_OBC_Temp'  initValue=0  dataType=double  storage=Volatile (RAM)  calVisible=on  calType=Measurement  calDispType=Number  calEnum={'False', 'True'}  calGain=1.0  calOffset=0  calMin=-inf  calMax=inf  calFormat='-1'  calUnit=''  calHelp=''  calAccess=1  calFunction=raptor_xcp_function(gcb)  calDispHeaders=off  calColHeaders={'Col1' 'Col2' 'Col3'}  calRowHeaders={'Row1' 'Row2' 'Row3'}
      settings: SourceProductName=Raptor
  raptor_data_write3 : Raptor_lib/Data Storage/raptor_data_write  dataName='Read_OBC_Status'  dataShape=Scalar  idxSource=Input Port  idxRow=1  idxCol=1
      settings: SourceProductName=Raptor
  raptor_data_write6 : Raptor_lib/Data Storage/raptor_data_write  dataName='Read_OBC_Temp'  dataShape=Scalar  idxSource=Input Port  idxRow=1  idxCol=1
      settings: SourceProductName=Raptor
  raptor_data_write7 : Raptor_lib/Data Storage/raptor_data_write  dataName='OBC_Age'  dataShape=Scalar  idxSource=Input Port  idxRow=1  idxCol=1
      settings: SourceProductName=Raptor
  raptor_data_write8 : Raptor_lib/Data Storage/raptor_data_write  dataName='Read_OBC_Vout'  dataShape=Scalar  idxSource=Input Port  idxRow=1  idxCol=1
      settings: SourceProductName=Raptor
  raptor_data_write9 : Raptor_lib/Data Storage/raptor_data_write  dataName='Read_OBC_Cout'  dataShape=Scalar  idxSource=Input Port  idxRow=1  idxCol=1
      settings: SourceProductName=Raptor
  raptor_measurement : Raptor_lib/Data Storage/raptor_measurement  paramName='Meas_OBC_ID'  nameSource=Parameter  calDispType=Number  calEnum={'False', 'True'}  calGain=1.0  calOffset=0.0  calMax=inf  calMin=-inf  calFormat='-1'  calUnit=''  calHelp=''  calAccess=1  calFunction=raptor_xcp_function(gcb)  calVisible=on
      settings: SourceProductName=Raptor
  wires:
  Demux/5 -> Data Type Conversion1/1
  Constant2/1 -> Convert_Byte2Data2/4(Factor)
  raptor_can_rxraw/5 -> Demux/1
  Demux/1 -> Convert_Byte2Data3/1(HighByte)
  Demux/3 -> Convert_Byte2Data1/1(HighByte)
  Constant/1 -> Convert_Byte2Data3/4(Factor), Convert_Byte2Data1/4(Factor)
  Demux/2 -> Convert_Byte2Data3/2(LowByte)
  Convert_Byte2Data3/1(Data) -> Mux/1
  Convert_Byte2Data1/1(Data) -> Mux/2
  raptor_can_rxraw/1 -> raptor_data_write7/1
  Demux1/2 -> raptor_data_write9/1
  Data Type Conversion1/1 -> Mux/3
  Demux/4 -> Convert_Byte2Data1/2(LowByte)
  Data Type Conversion/1 -> raptor_data_write3/1
  Mux/1 -> Demux1/1
  Demux1/3 -> Data Type Conversion/1
  Demux1/4 -> raptor_data_write6/1
  Constant1/1 -> Convert_Byte2Data2/3(Offset)
  Demux1/1 -> raptor_data_write8/1
  Convert_Byte2Data2/1(Data) -> Mux/4
  Demux/6 -> Convert_Byte2Data2/2(LowByte)
  raptor_can_rxraw/3 -> raptor_measurement/1

== system EPT/Foreground_TimeBase_5ms/CAN/CAN3_exec/OBC/OBC/OBC_Tx ==
  Trigger : TriggerPort  VariantControl=Variant  PortDimensions=1
  Constant : Constant  OutDataTypeStr=boolean
  Constant1 : Constant  Value=8  OutDataTypeStr=uint8
  Constant2 : Constant  Value=0.1
  Convert_Data2Byte : Subsystem
  Convert_Data2Byte1 : Subsystem
  Data Type Conversion{,1..5} (6 alike) : DataTypeConversion  OutDataTypeStr=uint8
  Mux : Mux  Inputs=8
  raptor_adjustment : Raptor_lib/Data Storage/raptor_adjustment  paramName='Cal_OBC_TxID'  nameSource=Parameter  initValue=hex2dec('1801E5F4')  dataType=uint32  storage=Calibration  calDispType=Number  calEnum={'False', 'True'}  calGain=1.0  calOffset=0.0  calMax=inf  calMin=-inf  calFormat='-1'  calUnit=''  calHelp=''  calAccess=1  calFunction=raptor_xcp_function(gcb)  calDispHeaders=off  calColHeaders={'Col1' 'Col2' 'Col3'}  calRowHeaders={'Row1' 'Row2' 'Row3'}
      settings: SourceProductName=Raptor
  raptor_can_txraw : Raptor_lib/CAN/raptor_can_txraw  canBus='CAN3'  queueSize=1  showIdTypePort=1  idTypeSelectValues=Standard|Extended  idTypeSelect=Standard
      settings: SourceProductName=Raptor
  raptor_data_def1 : Raptor_lib/Data Storage/raptor_data_def  dataName='EPT_OBC_VOUT_CMD'  initValue=110  dataType=double  storage=Volatile (RAM)  calVisible=on  calType=Measurement  calDispType=Number  calEnum={'False', 'True'}  calGain=1.0  calOffset=0  calMin=-inf  calMax=inf  calFormat='-1'  calUnit=''  calHelp=''  calAccess=1  calFunction=raptor_xcp_function(gcb)  calDispHeaders=off  calColHeaders={'Col1' 'Col2' 'Col3'}  calRowHeaders={'Row1' 'Row2' 'Row3'}
      settings: SourceProductName=Raptor
  raptor_data_def4 : Raptor_lib/Data Storage/raptor_data_def  dataName='EPT_OBC_IOUT_CMD'  initValue=0  dataType=double  storage=Volatile (RAM)  calVisible=on  calType=Measurement  calDispType=Number  calEnum={'False', 'True'}  calGain=1.0  calOffset=0  calMin=-inf  calMax=inf  calFormat='-1'  calUnit=''  calHelp=''  calAccess=1  calFunction=raptor_xcp_function(gcb)  calDispHeaders=off  calColHeaders={'Col1' 'Col2' 'Col3'}  calRowHeaders={'Row1' 'Row2' 'Row3'}
      settings: SourceProductName=Raptor
  raptor_data_def6 : Raptor_lib/Data Storage/raptor_data_def  dataName='EPT_OBC_EN'  initValue=0  dataType=uint8  storage=Volatile (RAM)  calVisible=on  calType=Measurement  calDispType=Number  calEnum={'False', 'True'}  calGain=1.0  calOffset=0  calMin=-inf  calMax=inf  calFormat='-1'  calUnit=''  calHelp=''  calAccess=1  calFunction=raptor_xcp_function(gcb)  calDispHeaders=off  calColHeaders={'Col1' 'Col2' 'Col3'}  calRowHeaders={'Row1' 'Row2' 'Row3'}
      settings: SourceProductName=Raptor
  raptor_data_def7 : Raptor_lib/Data Storage/raptor_data_def  dataName='EPT_OBC_STA'  initValue=0  dataType=uint8  storage=Volatile (RAM)  calVisible=on  calType=Measurement  calDispType=Number  calEnum={'False', 'True'}  calGain=1.0  calOffset=0  calMin=-inf  calMax=inf  calFormat='-1'  calUnit=''  calHelp=''  calAccess=1  calFunction=raptor_xcp_function(gcb)  calDispHeaders=off  calColHeaders={'Col1' 'Col2' 'Col3'}  calRowHeaders={'Row1' 'Row2' 'Row3'}
      settings: SourceProductName=Raptor
  raptor_data_read3 : Raptor_lib/Data Storage/raptor_data_read  dataName='EPT_OBC_VOUT_CMD'  dataShape=Scalar  idxSource=Input  idxRow=1  idxCol=1
      settings: SourceProductName=Raptor
  raptor_data_read4 : Raptor_lib/Data Storage/raptor_data_read  dataName='EPT_OBC_IOUT_CMD'  dataShape=Scalar  idxSource=Input  idxRow=1  idxCol=1
      settings: SourceProductName=Raptor
  raptor_data_read6 : Raptor_lib/Data Storage/raptor_data_read  dataName='EPT_OBC_EN'  dataShape=Scalar  idxSource=Input  idxRow=1  idxCol=1
      settings: SourceProductName=Raptor
  raptor_data_read7 : Raptor_lib/Data Storage/raptor_data_read  dataName='EPT_OBC_STA'  dataShape=Scalar  idxSource=Input  idxRow=1  idxCol=1
      settings: SourceProductName=Raptor
  raptor_override : Raptor_lib/Data Storage/raptor_override  paramName='Cal_OBC_Current'  nameSource=Parameter  measurement=None  calDispType=Number  calEnum={'False', 'True'}  calGain=1.0  calOffset=0.0  calMax=inf  calMin=-inf  calFormat='-1'  calUnit=''  calHelp=''  calAccess=1  calFunction=[raptor_xcp_function(gcb) '|' raptor_get_param_eval(gcb, 'paramName') '_Override']
      settings: SourceProductName=Raptor
  raptor_override1 : Raptor_lib/Data Storage/raptor_override  paramName='Cal_OBC_Voltage'  nameSource=Parameter  measurement=None  calDispType=Number  calEnum={'False', 'True'}  calGain=1.0  calOffset=0.0  calMax=inf  calMin=-inf  calFormat='-1'  calUnit=''  calHelp=''  calAccess=1  calFunction=[raptor_xcp_function(gcb) '|' raptor_get_param_eval(gcb, 'paramName') '_Override']
      settings: SourceProductName=Raptor
  raptor_override2 : Raptor_lib/Data Storage/raptor_override  paramName='Cal_OBC_EN'  nameSource=Parameter  measurement=None  calDispType=Number  calEnum={'False', 'True'}  calGain=1.0  calOffset=0.0  calMax=inf  calMin=-inf  calFormat='-1'  calUnit=''  calHelp=''  calAccess=1  calFunction=[raptor_xcp_function(gcb) '|' raptor_get_param_eval(gcb, 'paramName') '_Override']
      settings: SourceProductName=Raptor
  raptor_override3 : Raptor_lib/Data Storage/raptor_override  paramName='Cal_OBC_Status'  nameSource=Parameter  measurement=None  calDispType=Number  calEnum={'False', 'True'}  calGain=1.0  calOffset=0.0  calMax=inf  calMin=-inf  calFormat='-1'  calUnit=''  calHelp=''  calAccess=1  calFunction=[raptor_xcp_function(gcb) '|' raptor_get_param_eval(gcb, 'paramName') '_Override']
      settings: SourceProductName=Raptor
  wires:
  Convert_Data2Byte/1(HighByte) -> Data Type Conversion/1
  Constant1/1 -> raptor_can_txraw/3
  Convert_Data2Byte1/1(HighByte) -> Data Type Conversion2/1
  Data Type Conversion2/1 -> Mux/3
  Constant2/1 -> Convert_Data2Byte1/2(Factor), Convert_Data2Byte/2(Factor)
  Data Type Conversion5/1 -> Mux/6
  raptor_adjustment/1 -> raptor_can_txraw/2
  raptor_data_read6/1 -> raptor_override2/1
  Data Type Conversion4/1 -> Mux/5
  Data Type Conversion1/1 -> Mux/2
  Data Type Conversion3/1 -> Mux/4
  Data Type Conversion/1 -> Mux/1
  Convert_Data2Byte/2(LowByte) -> Data Type Conversion1/1
  raptor_override3/1 -> Data Type Conversion5/1
  raptor_override/1 -> Convert_Data2Byte1/1(Data)
  raptor_override2/1 -> Data Type Conversion4/1
  raptor_override1/1 -> Convert_Data2Byte/1(Data)
  Mux/1 -> raptor_can_txraw/4
  raptor_data_read4/1 -> raptor_override/1
  Constant/1 -> raptor_can_txraw/1
  raptor_data_read7/1 -> raptor_override3/1
  raptor_data_read3/1 -> raptor_override1/1
  Convert_Data2Byte1/2(LowByte) -> Data Type Conversion3/1

== system EPT/Foreground_TimeBase_5ms/CAN/CAN3_exec/PWCU_GENERATOR/CountTrigger/CycleTrigger ==
  In1 : Inport
  In2 : Inport  Port=2
  Add : Sum
  Add1 : Sum
  Add2 : Sum  Inputs=+-
  Constant1 : Constant
  Constant2 : Constant  Value=0
  Constant3 : Constant
  Data Type Conversion1 : DataTypeConversion
  Data Type Conversion2 : DataTypeConversion
  Display : Display
  Relational Operator1 : RelationalOperator  OutDataTypeStr=boolean  RndMeth=Simplest
  Scope : Scope
  Scope1 : Scope
  Scope2 : Scope
  Switch : Switch  Threshold=1
  Unit Delay : UnitDelay  SampleTime=-1  HasFrameUpgradeWarning=on
  Unit Delay1 : UnitDelay  SampleTime=-1  HasFrameUpgradeWarning=on
  Trigger : Outport  VectorParamsAs1DForOutWhenUnconnected=off
  wires:
  Constant3/1 -> Add2/2
  In2/1 -> Add2/1
  Add2/1 -> Data Type Conversion1/1
  Data Type Conversion2/1 -> Switch/2, Add/2
  Constant2/1 -> Switch/3
  Data Type Conversion1/1 -> Relational Operator1/2
  Relational Operator1/1 -> Trigger/1, Scope2/1
  Constant1/1 -> Add1/2
  Unit Delay1/1 -> Add1/1
  Add1/1 -> Display/1, Unit Delay1/1, Scope/1
  Switch/1 -> Unit Delay/1, Scope1/1, Relational Operator1/1
  Unit Delay/1 -> Add/1
  In1/1 -> Data Type Conversion2/1
  Add/1 -> Switch/1

== system EPT/Foreground_TimeBase_5ms/CAN/CAN3_exec/PWCU_GENERATOR/CountTrigger1/CycleTrigger ==
  In1 : Inport
  In2 : Inport  Port=2
  Add : Sum
  Add1 : Sum
  Add2 : Sum  Inputs=+-
  Constant1 : Constant
  Constant2 : Constant  Value=0
  Constant3 : Constant
  Data Type Conversion1 : DataTypeConversion
  Data Type Conversion2 : DataTypeConversion
  Display : Display
  Relational Operator1 : RelationalOperator  OutDataTypeStr=boolean  RndMeth=Simplest
  Scope : Scope
  Scope1 : Scope
  Scope2 : Scope
  Switch : Switch  Threshold=1
  Unit Delay : UnitDelay  SampleTime=-1  HasFrameUpgradeWarning=on
  Unit Delay1 : UnitDelay  SampleTime=-1  HasFrameUpgradeWarning=on
  Trigger : Outport  VectorParamsAs1DForOutWhenUnconnected=off
  wires:
  Constant3/1 -> Add2/2
  In2/1 -> Add2/1
  Add2/1 -> Data Type Conversion1/1
  Data Type Conversion2/1 -> Switch/2, Add/2
  Constant2/1 -> Switch/3
  Data Type Conversion1/1 -> Relational Operator1/2
  Relational Operator1/1 -> Trigger/1, Scope2/1
  Constant1/1 -> Add1/2
  Unit Delay1/1 -> Add1/1
  Add1/1 -> Display/1, Unit Delay1/1, Scope/1
  Switch/1 -> Unit Delay/1, Scope1/1, Relational Operator1/1
  Unit Delay/1 -> Add/1
  In1/1 -> Data Type Conversion2/1
  Add/1 -> Switch/1
